simulink model "TesteRede"  (Simulink 8.5)
settings: Solver=ode23tb  StartTime=0.0  StopTime=3  FixedStep=1e-4  MaxStep=1e-3  RelTol=1e-3
libraries: powerlib x13, AvgModels x3, powerlib_meascontrol x2
settings Model: Creator=Batlab  LastModifiedBy=lgalo
settings OptimizationCC: InitFltsAndDblsToZero=on
settings DebuggingCC: SaveWithParameterizedLinksMsg=none  SolverPrmCheckMsg=warning  FcnCallInpInsideContextMsg=UseLocalSettings
settings GRTTargetCC: TargetFcnLib=ansi_tfl_tmw.mat

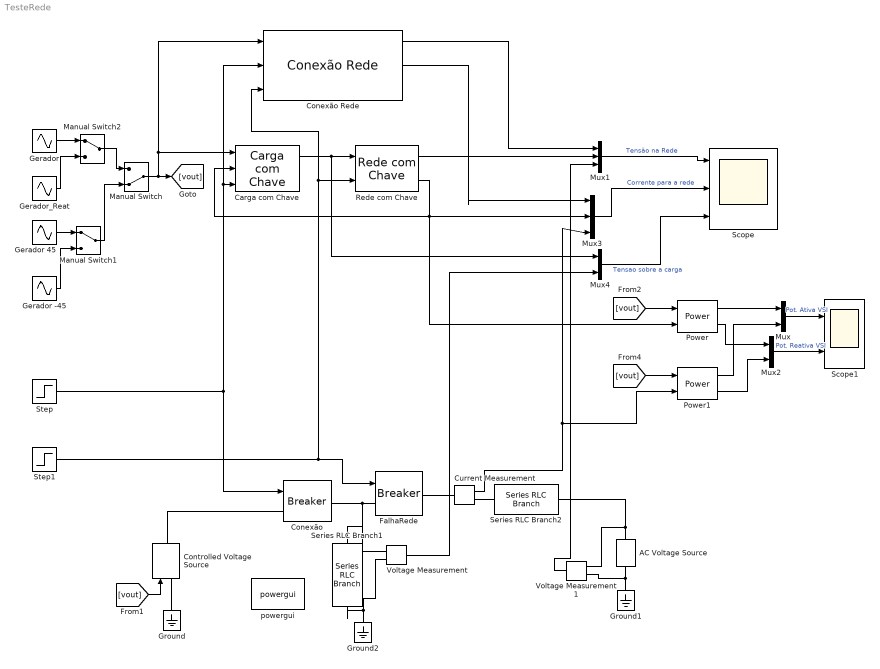
== system TesteRede ==
  AC Voltage Source : powerlib/Electrical Sources/AC Voltage Source  Amplitude=181  Phase=0  Frequency=60  SampleTime=0  Measurements=None
  Carga com Chave : AvgModels/Carga com Chave  Rl=10  Rsmin=0.1  Rsmax=1e6
  Conexão : powerlib/Elements/Breaker  InitialState=0  SwitchingTimes="[1/60  5/60]"  External=on  BreakerResistance=0.01  SnubberResistance=1e6  SnubberCapacitance=inf  Measurements=None  MoreParameters=on  NoBreakLoop=off
  Conexão Rede : AvgModels/Conexão Rede  Lg=10e-3  Rg=0.1  Vrede=127  frede=60  Rl=10  Rsmin=0.1  Rsmax=1e6
  Controlled Voltage Source : powerlib/Electrical Sources/Controlled Voltage Source  Initialize=on  Source_Type=AC  Amplitude=127  Phase=0  Frequency=60  Measurements=None
  Current Measurement : powerlib/Measurements/Current Measurement  PhasorSimulation=off  OutputType=Complex  PSBequivalent=0
  FalhaRede : powerlib/Elements/Breaker  InitialState=1  SwitchingTimes=[2]  External=on  BreakerResistance=0.01  SnubberResistance=1e6  SnubberCapacitance=inf  Measurements=None  MoreParameters=on  NoBreakLoop=off
  Gerador : Sin  Amplitude=127*sqrt(2)  Frequency=60*2*pi  SampleTime=0
  Gerador -45 : Sin  Amplitude=127*sqrt(2)  Frequency=60*2*pi  Phase=-pi/4  SampleTime=0
  Gerador 45 : Sin  Amplitude=127*sqrt(2)  Frequency=60*2*pi  Phase=pi/12  SampleTime=0
  Gerador_Reat : Sin  Amplitude=127*sqrt(2)+10  Frequency=60*2*pi  SampleTime=0
  Ground : powerlib/Elements/Ground  LConnTagsString=a
  Ground1 : powerlib/Elements/Ground  LConnTagsString=a
  Ground2 : powerlib/Elements/Ground  LConnTagsString=a
  Manual Switch : ManualSwitch  CurrentSetting=0
  Manual Switch1 : ManualSwitch
  Manual Switch2 : ManualSwitch
  Mux : Mux  Inputs=2
  Mux1 : Mux  Inputs=3
  Mux2 : Mux  Inputs=2
  Mux3 : Mux  Inputs=3
  Mux4 : Mux  Inputs=2
  Power : powerlib_meascontrol/Measurements/Power  Freq=60  Vinit=[1, 0]  Iinit=[1, 0]  Ts=0
  Power1 : powerlib_meascontrol/Measurements/Power  Freq=60  Vinit=[1, 0]  Iinit=[1, 0]  Ts=0
  Rede com Chave : AvgModels/Rede com Chave  Lg=10e-3  Rg=0.1  Vrede=127  frede=60  Rsmin=0.01  Rsmax=1e6
  Scope : Scope  NumInputPorts=3
      settings: TimeRange=3  YMin=-200~-20~-1500  YMax=200~20~1500  SaveName=dados
  Scope1 : Scope  NumInputPorts=2
      settings: TimeRange=3  YMin=-1500~-1200  YMax=1500~400  SaveName=dados1
  Series RLC Branch1 : powerlib/Elements/Series RLC Branch  LConnTagsString=__new0  RConnTagsString=__new0  BranchType=R  Resistance=10  Inductance=10e-3  SetiL0=off  InitialCurrent=0  Capacitance=1e-6  Setx0=off  InitialVoltage=0  Measurements=None
  Series RLC Branch2 : powerlib/Elements/Series RLC Branch  LConnTagsString=__new0  RConnTagsString=__new0  BranchType=RL  Resistance=0.1  Inductance=10e-3  SetiL0=off  InitialCurrent=0  Capacitance=1e-6  Setx0=off  InitialVoltage=0  Measurements=None
  Step : Step  SampleTime=0
  Step1 : Step  Time=2  Before=1  After=0  SampleTime=0
  Voltage Measurement : powerlib/Measurements/Voltage Measurement  PhasorSimulation=off  OutputType=Complex  PSBequivalent=0
  Voltage Measurement1 : powerlib/Measurements/Voltage Measurement  PhasorSimulation=off  OutputType=Complex  PSBequivalent=0
  powergui : powerlib/powergui  Priority=1  SimulationMode=Continuous  SolverType=Tustin/Backward Euler (TBE)  SampleTime=50e-6  frequency=60  SPID=off  DisableSnubberDevices=off  DisableRonSwitches=off  DisableVfSwitches=off  SwTol=0  DisplayEquations=off  Interpol=off  methode=off  Ts=100  FunctionMessages=off  echomessages=off  HookPort=off  EnableUseOfTLC=off  x0status=blocks  frequencyindice=60  Pbase=100e6  ErrMax=1e-4  Iterations=50  UnitsV=kV  UnitsW=MW  buscounter=0  RestoreLinks=warning  ResistiveCurrentMeasurement=off  Frange=[0:2:500]  Ylog=off  Xlog=on  ShowGrid=off  save=off  variable=ZData  structure=0  ZoomFFT=off  StartTime=0.0  cycles=1  DisplayStyle=1  fundamental=60  FreqAxis=off  MaxFrequency=1000  frequencyindicesteady=1  RmsSteady=1  display=off
  wires:
  Power/2 -> Mux2/1
  Power/1 -> Mux/1
  Mux/1 -> Scope1/1  "Pot. Ativa VSI"
  Step/1 -> Conexão Rede/2, Carga com Chave/3, Conexão/1
  Gerador 45/1 -> Manual Switch1/1
  Manual Switch1/1 -> Manual Switch/2
  Gerador -45/1 -> Manual Switch1/2
  Gerador/1 -> Manual Switch2/1
  Manual Switch2/1 -> Manual Switch/1
  Gerador_Reat/1 -> Manual Switch2/2
  Manual Switch/1 -> Conexão Rede/1, Carga com Chave/1, [vout]
  [vout] -> Controlled Voltage Source/1
  [vout] -> Power/1
  Current Measurement/1 -> Mux3/3, Power1/2
  [vout] -> Power1/1
  Power1/1 -> Mux/2
  Step1/1 -> Conexão Rede/3, Rede com Chave/2, FalhaRede/1
  Mux2/1 -> Scope1/2  "Pot. Reativa VSI"
  Power1/2 -> Mux2/2
  Mux3/1 -> Scope/2  "Corrente para a rede"
  Rede com Chave/1 -> Mux1/2
  Rede com Chave/2 -> Mux3/2, Carga com Chave/2, Power/2
  Carga com Chave/1 -> Mux4/1, Rede com Chave/1
  Conexão Rede/1 -> Mux1/1
  Mux1/1 -> Scope/1  "Tensão na Rede"
  Conexão Rede/2 -> Mux3/1
  Voltage Measurement1/1 -> Mux1/3
  Voltage Measurement/1 -> Mux4/2
  Mux4/1 -> Scope/3  "Tensao sobre a carga"
  connections:
  Conexão/RConn1 -- Series RLC Branch1/LConn1 -- Voltage Measurement/LConn1 -- FalhaRede/LConn1
  Ground/LConn1 -- Controlled Voltage Source/LConn1
  Ground1/LConn1 -- Voltage Measurement1/LConn2 -- AC Voltage Source/LConn1
  Ground2/LConn1 -- Series RLC Branch1/RConn1 -- Voltage Measurement/LConn2
  Series RLC Branch2/RConn1 -- Voltage Measurement1/LConn1 -- AC Voltage Source/RConn1
  FalhaRede/RConn1 -- Current Measurement/LConn1
  Current Measurement/RConn1 -- Series RLC Branch2/LConn1
  Controlled Voltage Source/RConn1 -- Conexão/LConn1
